simulink model "Divide_Integer"  (R2017b)
settings: Solver=ode3  StartTime=0.0  StopTime=10.0  FixedStep=0.200000  RelTol=1e-3
settings Model: Creator=hbourbou  LastModifiedBy=hbourbou
settings OptimizationCC: LifeSpan=inf
settings DebuggingCC: SFExecutionAtInitializationDiag=none
settings HardwareCC: ProdBitPerSizeT=32  ProdBitPerPtrDiffT=32  ProdWordSize=32  ProdHWDeviceType=Specified
settings CodeAppCC: StateflowObjectComments=on

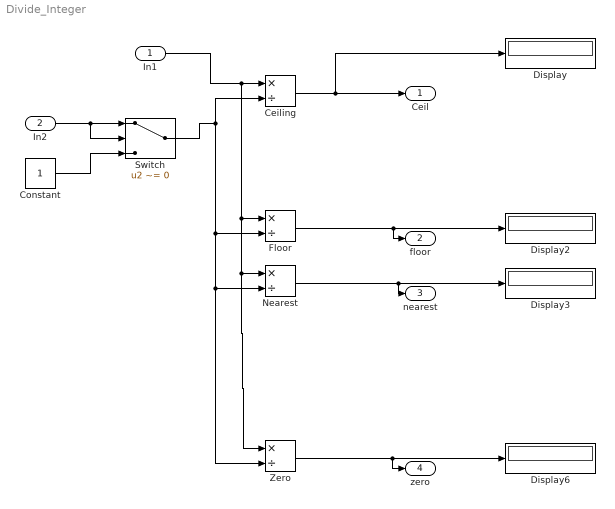
== system Divide_Integer ==
  In1 : Inport  OutDataTypeStr=int8
  In2 : Inport  Port=2  OutDataTypeStr=int8
  Ceiling : Product  Inputs=*/  RndMeth=Ceiling
  Constant : Constant  OutDataTypeStr=int8
  Display{,2..3,6} (4 alike) : Display
  Floor : Product  Inputs=*/
  Nearest : Product  Inputs=*/  RndMeth=Nearest
  Switch : Switch  Criteria=u2 ~= 0
  Zero : Product  Inputs=*/  RndMeth=Zero
  Ceil : Outport
  floor : Outport  Port=2
  nearest : Outport  Port=3
  zero : Outport  Port=4
  wires:
  Switch/1 -> Zero/2, Nearest/2, Floor/2, Ceiling/2
  In1/1 -> Zero/1, Nearest/1, Floor/1, Ceiling/1
  Ceiling/1 -> Ceil/1, Display/1
  Floor/1 -> floor/1, Display2/1
  Nearest/1 -> nearest/1, Display3/1
  Zero/1 -> zero/1, Display6/1
  In2/1 -> Switch/1, Switch/2
  Constant/1 -> Switch/3
